simulink model "parent_model_v2"  (R2020b)
settings: Solver=VariableStepAuto  StartTime=0.0  StopTime=10.0  RelTol=1e-3
libraries: sdl_lib x14, nesl_utility x12, autolibmappedmotor x4, autolibdatasheetbattery x1, autolibshared x1
settings Model: Creator=True  LastModifiedBy=True

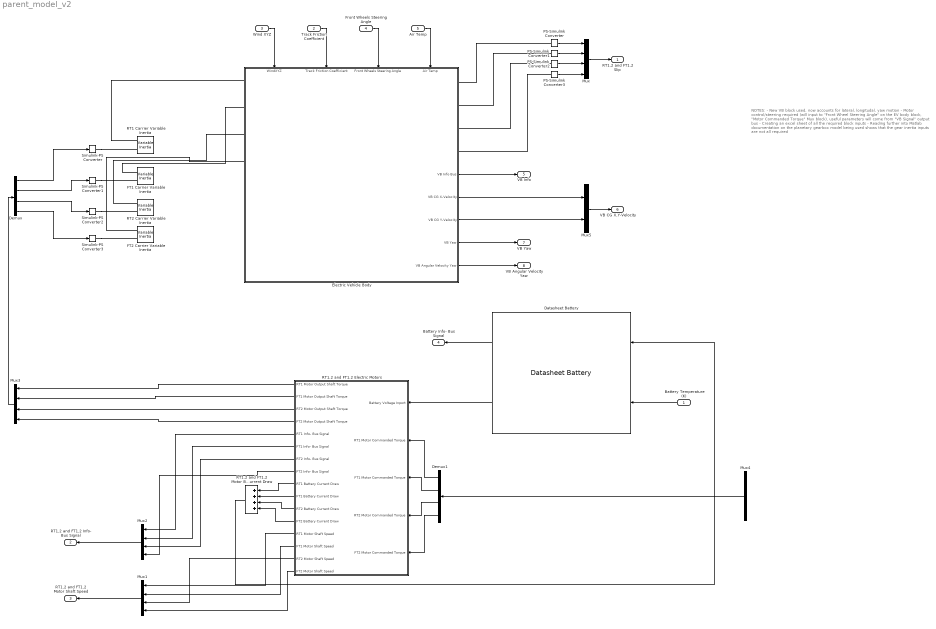
== system parent_model_v2 ==
  note: NOTES:
      | - New VB block used, now accounts for lateral, longitudal, yaw motion
      |
      | - Motor control/steering required (will input to "Front Wheel Steering Angle" on the EV body block, "Motor Commanded Torque" Mux block), useful parameters will come from "VB Signal" output bus
      |
      | - Creating an excel sheet of all the required block inputs
      |
      | - Reading further into Matlab documentation on the planetary gearbox model being used shows that the gear inertia inputs are not all required
  Battery Temperature (K) : Inport
  Track Friction Coefficient : Inport  Port=2
  Wind XYZ : Inport  Port=3
  Front Wheels Steering Angle : Inport  Port=4
  Air Temp : Inport  Port=5
  Datasheet Battery : autolibdatasheetbattery/Datasheet Battery  CapacityCtrl=Parameter  OutputVlt=Unfiltered  BattChargeMax=100  Em=[2.8 3.228 3.284 3.361 3.408 3.427 3.472 3.477 3.493 3.504 3.516 3.528 3.537 3.545 3.555 3.561 3.566 3.576 3.587 3.589 3.594 3.6 3.608 3.61 3.616 3.619 3.626 3.632 3.637 3.64 3.645 3.646 3.652 3.655 3.658 3.661 3.664 3.668 3.673 3.678 3.68 3.681 3.686 3.692 3.699 3.702 3.705 3.71 3.717 3.723 3.728 3.733 3.735 3.742 3.749 3.755 3.761 3.768 3.773 3.78 3.791 3.798 3.798 3.814 3.818 3.825 3.841 3.846 3.855 3.863 3.877 3.885 3.894 3.907 3.919 3.926 3.935 3.944 3.954 3.964 3.974 3.988 3.998 4.014 4.029 4.034 4.047 4.065 4.074 4.086 4.097 4.131 4.126 4.138 4.15 4.18 4.174 4.187 4.207 4.231 4.221]  CapLUTBp=[0 0.01 0.02 0.03 0.04 0.05 0.06 0.07 0.08 0.09 0.1 0.11 0.12 0.13 0.14 0.15 0.16 0.17 0.18 0.19 0.2 0.21 0.22 0.23 0.24 0.25 0.26 0.27 0.28 0.29 0.3 0.31 0.32 0.33 0.34 0.35 0.36 0.37 0.38 0.39 0.4 0.41 0.42 0.43 0.44 0.45 0.46 0.47 0.48 0.49 0.5 0.51 0.52 0.53 0.54 0.55 0.56 0.57 0.58 0.59 0.6 0.61 0.62 0.63 0.64 0.65 0.66 0.67 0.68 0.69 0.7 0.71 0.72 0.73 0.74 0.75 0.76 0.77 0.78 0.79 0.8 0.81 0.82 0.83 0.84 0.85 0.86 0.87 0.88 0.89 0.9 0.91 0.92 0.93 0.94 0.95 0.96 0.97 0.98 0.99 1]  RInt=[0.008846 0.009319 0.009027 0.00847 0.01032 0.01314;0.006389 0.006554 0.005553 0.005525 0.006043 0.007805;0.004364 0.004101 0.00406 0.003452 0.003846 0.004517;0.002031 0.002563 0.002532 0.00246 0.002716 0.003047;0.001443 0.001825 0.001795 0.001778 0.001924 0.002234;0.0005603 0.0007192 0.0006887 0.0007557 0.0007355 0.001014;0.001028 0.001338 0.001 0.001536 0.001546 0.002789]  BattTempBp=[243.1 253.1 263.1 273.1 283.1 298.1 313.1]  CapSOCBp=[0 0.2 0.4 0.6 0.8 1]  Ns=1  Np=1  BattCapInit=100  Tc=1/1000  Vinit=4.221  RefBlkName='autolibdatasheetbattery/Datasheet Battery'
      settings: SourceProductBaseCode=PW
  Demux : Demux
  Demux1 : Demux
  Electric Vehicle Body : Subsystem
      settings: PortSchema="{\"entries\":[{\"content\":{\"sides\":[{\"content\":{\"connectorIds\":[\"LConn1\",\"LConn2\",\"LConn3\",\"LConn4\",\"LConn5\",\"LConn6\",\"LConn7\",\"LConn8\"]},\"type\":\"ConnectorPlacement.EquallySpacedRectSide\",\"uuid\":\"3589ffd8-3282-449f-9f73-db5573b89272\"},{\"content\":{\"connectorIds\":[\"RConn1\",\"RConn2\",\"RConn3\",\"RConn4\",\"Out1\",\"Out2\",\"Out3\",\"Out4\",\"Out5\"],\"side\":\"RIGHT\"},\"type\":\"ConnectorPlacement.EquallySpacedRectSide\",\"uuid\":\"4bc75fc4-5a6d-4cdc-a1d8-7589f1bfd0e3\"},{\"content\":{\"connectorIds\":[\"In1\",\"In2\",\"In3\",\"In4\"],\"side\":\"TOP\"},\"type\":\"ConnectorPlacement.EquallySpacedRectSide\",\"uuid\":\"5582f31c-489d-4354-9c03-0beb1d144974\"},{\"content\":{\"connectorIds\":[],\"side\":\"BOTTOM\"},\"type\":\"ConnectorPlacement.EquallySpacedRectSide\",\"uuid\":\"e952a40a-921b-4756-bc3d-1bba2f446a83\"},{\"content\":{\"connectorIds\":[],\"side\":\"HIDDEN\"},\"type\":\"ConnectorPlacement.EquallySpacedRectSide\",\"uuid\":\"95051cab-6025-4def-8e94-855365c64cfc\"}]},\"type\":\"ConnectorPlacement.EquallySpacedConnector\",\"uuid\":\"f0af1aeb-7bbe-491f-85c8-fb0f3026e409\"}],\"packageUris\":[\"http://schema.mathworks.com/mf0/Connector/R2020b\"],\"version\":\"1.0\"}"
  FT1 Carrier Variable Inertia : sdl_lib/Inertias & Loads/Variable Inertia  minimum_inertia=0.1 kg*m^2  L_specify=off  L_priority=High  L=0 m^2*kg/s  L_nominal_specify=off  L_nominal_unit=m^2*kg/s  L_nominal_value=1
      settings: SourceProductBaseCode=LD  InternalSimscapePortConfiguration="{\"Bottom\":[],\"Left\":[{\"id\":\"I\",\"label\":\"\",\"type\":\"input\"},{\"id\":\"A\",\"label\":\"\",\"type\":\"foundation.mechanical.rotational.rotational\"}],\"Right\":[],\"Top\":[]}"
  FT2 Carrier Variable Inertia : sdl_lib/Inertias & Loads/Variable Inertia  minimum_inertia=0.1 kg*m^2  L_specify=off  L_priority=High  L=0 m^2*kg/s  L_nominal_specify=off  L_nominal_unit=m^2*kg/s  L_nominal_value=1
      settings: SourceProductBaseCode=LD  InternalSimscapePortConfiguration="{\"Bottom\":[],\"Left\":[{\"id\":\"I\",\"label\":\"\",\"type\":\"input\"},{\"id\":\"A\",\"label\":\"\",\"type\":\"foundation.mechanical.rotational.rotational\"}],\"Right\":[],\"Top\":[]}"
  Mux{,1..4} (5 alike) : Mux
  Mux5 : Mux  Inputs=2
  PS-Simulink Converter{,1..3} (4 alike) : nesl_utility/PS-Simulink Converter  PhysicalDomain=network_engine_domain  SubClassName=ps_output  LeftPortType=input  RightPortType=output  PseudoPeriodic=off  Frequencies=[]  Unit=inherit  AffineConversion=off
  RT1 Carrier Variable Inertia : sdl_lib/Inertias & Loads/Variable Inertia  minimum_inertia=0.1 kg*m^2  L_specify=off  L_priority=High  L=0 m^2*kg/s  L_nominal_specify=off  L_nominal_unit=m^2*kg/s  L_nominal_value=1
      settings: SourceProductBaseCode=LD  InternalSimscapePortConfiguration="{\"Bottom\":[],\"Left\":[{\"id\":\"I\",\"label\":\"\",\"type\":\"input\"},{\"id\":\"A\",\"label\":\"\",\"type\":\"foundation.mechanical.rotational.rotational\"}],\"Right\":[],\"Top\":[]}"
  RT1,2 and FT1,2 Electric Motors : Subsystem
  RT1,2 and FT1,2 Motor Battery Current Draw : Sum  Inputs=++++
  RT2 Carrier Variable Inertia : sdl_lib/Inertias & Loads/Variable Inertia  minimum_inertia=0.1 kg*m^2  L_specify=off  L_priority=High  L=0 m^2*kg/s  L_nominal_specify=off  L_nominal_unit=m^2*kg/s  L_nominal_value=1
      settings: SourceProductBaseCode=LD  InternalSimscapePortConfiguration="{\"Bottom\":[],\"Left\":[{\"id\":\"I\",\"label\":\"\",\"type\":\"input\"},{\"id\":\"A\",\"label\":\"\",\"type\":\"foundation.mechanical.rotational.rotational\"}],\"Right\":[],\"Top\":[]}"
  Simulink-PS Converter{,1..3} (4 alike) : nesl_utility/Simulink-PS Converter  PhysicalDomain=network_engine_domain  SubClassName=ps_input  LeftPortType=input  RightPortType=output  PseudoPeriodic=off  Frequencies=[]  NoiseDistribution=none  NoiseParameters=[]  Unit=1  AffineConversion=off  FilteringAndDerivatives=provide  SimscapeFilterOrder=1  InputFilterTimeConstant=0.001  UdotUserProvided=0
  RT1,2 and FT1,2 Slip : Outport
  RT1,2 and FT1,2 Info- Bus Signal : Outport  Port=2
  RT1,2 and FT1,2 Motor Shaft Speed : Outport  Port=3
  Battery Info- Bus Signal : Outport  Port=4
  VB Info : Outport  Port=5
  VB CG X,Y-Velocity : Outport  Port=6
  VB Yaw : Outport  Port=7
  VB Angular Velocity Yaw : Outport  Port=8
  wires:
  Datasheet Battery/2 -> RT1,2 and FT1,2 Electric Motors/1(Battery Voltage Inport)
  RT1,2 and FT1,2 Electric Motors/9(RT1 Battery Current Draw) -> RT1,2 and FT1,2 Motor Battery Current Draw/1
  RT1,2 and FT1,2 Electric Motors/10(FT1 Battery Current Draw) -> RT1,2 and FT1,2 Motor Battery Current Draw/2
  RT1,2 and FT1,2 Electric Motors/11(RT2 Battery Current Draw) -> RT1,2 and FT1,2 Motor Battery Current Draw/3
  RT1,2 and FT1,2 Electric Motors/12(FT2 Battery Current Draw) -> RT1,2 and FT1,2 Motor Battery Current Draw/4
  RT1,2 and FT1,2 Motor Battery Current Draw/1 -> Datasheet Battery/1
  Battery Temperature (K)/1 -> Datasheet Battery/2
  PS-Simulink Converter/1 -> Mux/1
  PS-Simulink Converter1/1 -> Mux/2
  PS-Simulink Converter2/1 -> Mux/3
  PS-Simulink Converter3/1 -> Mux/4
  Mux/1 -> RT1,2 and FT1,2 Slip/1
  RT1,2 and FT1,2 Electric Motors/5(RT1 Info- Bus Signal) -> Mux2/1
  RT1,2 and FT1,2 Electric Motors/6(FT1 Info- Bus Signal) -> Mux2/2
  RT1,2 and FT1,2 Electric Motors/7(RT2 Info- Bus Signal) -> Mux2/3
  RT1,2 and FT1,2 Electric Motors/8(FT2 Info- Bus Signal) -> Mux2/4
  RT1,2 and FT1,2 Electric Motors/13(RT1 Motor Shaft Speed) -> Mux1/1
  RT1,2 and FT1,2 Electric Motors/14(FT1 Motor Shaft Speed) -> Mux1/2
  RT1,2 and FT1,2 Electric Motors/15(RT2 Motor Shaft Speed) -> Mux1/3
  RT1,2 and FT1,2 Electric Motors/16(FT2 Motor Shaft Speed) -> Mux1/4
  Mux2/1 -> RT1,2 and FT1,2 Info- Bus Signal/1
  Mux1/1 -> RT1,2 and FT1,2 Motor Shaft Speed/1
  Datasheet Battery/1 -> Battery Info- Bus Signal/1
  Demux/1 -> Simulink-PS Converter/1
  Demux/4 -> Simulink-PS Converter3/1
  Demux/3 -> Simulink-PS Converter2/1
  Demux/2 -> Simulink-PS Converter1/1
  RT1,2 and FT1,2 Electric Motors/1(RT1 Motor Output Shaft Torque) -> Mux3/1
  RT1,2 and FT1,2 Electric Motors/2(FT1 Motor Output Shaft Torque) -> Mux3/2
  RT1,2 and FT1,2 Electric Motors/3(RT2 Motor Output Shaft Torque) -> Mux3/3
  RT1,2 and FT1,2 Electric Motors/4(FT2 Motor Output Shaft Torque) -> Mux3/4
  Mux3/1 -> Demux/1
  Demux1/1 -> RT1,2 and FT1,2 Electric Motors/2(RT1 Motor Commanded Torque)
  Demux1/2 -> RT1,2 and FT1,2 Electric Motors/3("FT1 Motor Commanded Torque ")
  Demux1/3 -> RT1,2 and FT1,2 Electric Motors/4(RT2 Motor Commanded Torque)
  Demux1/4 -> RT1,2 and FT1,2 Electric Motors/5(FT2 Motor Commanded Torque)
  Mux4/1 -> Demux1/1
  Electric Vehicle Body/1(VB Info Bus) -> VB Info/1
  Electric Vehicle Body/2("VB CG X-Velocity ") -> Mux5/1
  Electric Vehicle Body/3(VB CG Y-Velocity) -> Mux5/2
  Mux5/1 -> VB CG X,Y-Velocity/1
  Electric Vehicle Body/4(VB Yaw) -> VB Yaw/1
  Electric Vehicle Body/5(VB Angular Velocity Yaw) -> VB Angular Velocity Yaw/1
  Track Friction Coefficient/1 -> Electric Vehicle Body/2(Track Friction Coefficient)
  Wind XYZ/1 -> Electric Vehicle Body/1(WindXYZ)
  Front Wheels Steering Angle/1 -> Electric Vehicle Body/3(Front Wheels Steering Angle)
  Air Temp/1 -> Electric Vehicle Body/4(Air Temp)
  connections:
  Simulink-PS Converter1/RConn1 -- FT1 Carrier Variable Inertia/LConn1
  Simulink-PS Converter2/RConn1 -- RT2 Carrier Variable Inertia/LConn1
  Simulink-PS Converter/RConn1 -- RT1 Carrier Variable Inertia/LConn1
  Simulink-PS Converter3/RConn1 -- FT2 Carrier Variable Inertia/LConn1
  PS-Simulink Converter/LConn1 -- Electric Vehicle Body/RConn1
  PS-Simulink Converter1/LConn1 -- Electric Vehicle Body/RConn2
  Electric Vehicle Body/LConn1 -- RT1 Carrier Variable Inertia/LConn2
  PS-Simulink Converter2/LConn1 -- Electric Vehicle Body/RConn3
  PS-Simulink Converter3/LConn1 -- Electric Vehicle Body/RConn4
  FT1 Carrier Variable Inertia/LConn2 -- Electric Vehicle Body/LConn2
  RT2 Carrier Variable Inertia/LConn2 -- Electric Vehicle Body/LConn3
  FT2 Carrier Variable Inertia/LConn2 -- Electric Vehicle Body/LConn4

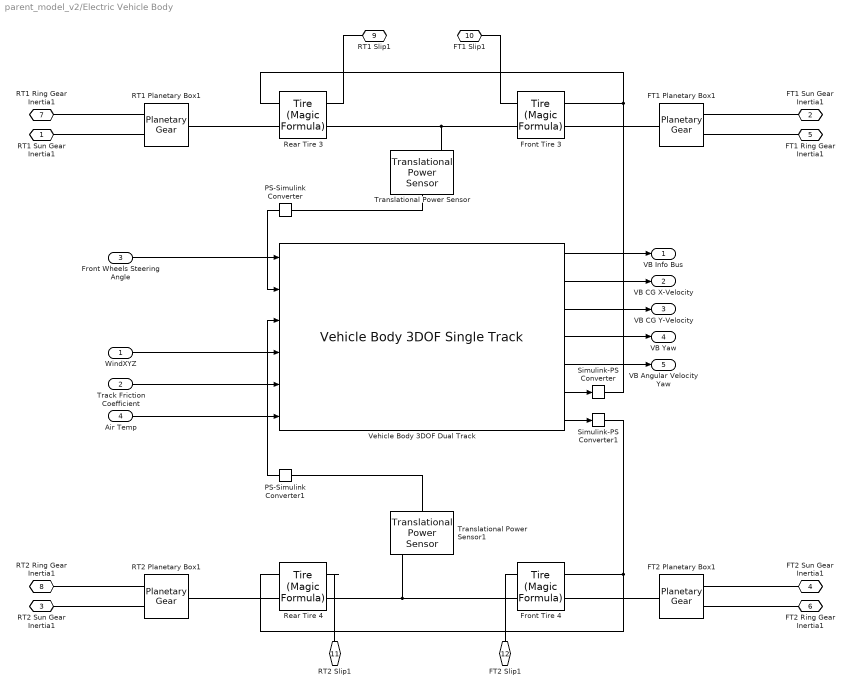
== system parent_model_v2/Electric Vehicle Body ==
  WindXYZ : Inport
  Track Friction Coefficient : Inport  Port=2
  Front Wheels Steering Angle : Inport  Port=3
  Air Temp : Inport  Port=4
  FT1 Planetary Box1 : sdl_lib/Gears/Planetary Gear  rs_ratio=2  friction_model=sdl.enum.gear_friction.none  mu_visc=[0, 0] N*m/(rad/s)  efficiency=[.96, .98]  temperature_TLU=[280, 300, 320] K  efficiency_sp_TLU=[.95, .9, .85]  efficiency_rp_TLU=[.95, .9, .85]  pwr_thr=[.001, .001] W  thermal_mass=50 J/K  T_init=300 K  model_inertia=simscape.enum.onoff.off  planet_inertia=0.001 kg*m^2
      settings: SourceProductBaseCode=LD
  FT2 Planetary Box1 : sdl_lib/Gears/Planetary Gear  rs_ratio=2  friction_model=sdl.enum.gear_friction.none  mu_visc=[0, 0] N*m/(rad/s)  efficiency=[.96, .98]  temperature_TLU=[280, 300, 320] K  efficiency_sp_TLU=[.95, .9, .85]  efficiency_rp_TLU=[.95, .9, .85]  pwr_thr=[.001, .001] W  thermal_mass=50 J/K  T_init=300 K  model_inertia=simscape.enum.onoff.off  planet_inertia=0.001 kg*m^2
      settings: SourceProductBaseCode=LD
  Front Tire 3 : sdl_lib/Tires & Vehicles/Tire (Magic Formula)  parameterization=sdl.enum.magic_tire_model.peak  F_z1=3000 N  F_x1=3500 N  kappa1=10  B_m=10  C_m=1.9  D_m=1  E_m=0.97  fz0=4000 N  p_Cx=1.685  p_Dx=[1.21, -.037]  p_Ex=[.344, .095, -.02, 0]  p_Kx=[21.51, -.163, .245]  p_Hx=[-.002, .002]  p_Vx=[0, 0]  v_tr_thr=0.1 m/s  r_e=0.3 m  model_compliance=0  stiffness=1e6 N/m  damping=1000 N/(m/s)  model_inertia=0  inertia=1 kg*m^2  initial_velocity=0 rad/s  model_resistance=0  resistance_model=1  coeff=0.015  p_tire=250e3 Pa  alpha=-0.003  beta=0.97  coeff_a=84e-4  coeff_b=6.2e-4 s/m  coeff_c=1.6e-4 s^2/m^2  v_thr=0.001 m/s
  Front Tire 4 : sdl_lib/Tires & Vehicles/Tire (Magic Formula)  parameterization=sdl.enum.magic_tire_model.peak  F_z1=3000 N  F_x1=3500 N  kappa1=10  B_m=10  C_m=1.9  D_m=1  E_m=0.97  fz0=4000 N  p_Cx=1.685  p_Dx=[1.21, -.037]  p_Ex=[.344, .095, -.02, 0]  p_Kx=[21.51, -.163, .245]  p_Hx=[-.002, .002]  p_Vx=[0, 0]  v_tr_thr=0.1 m/s  r_e=0.3 m  model_compliance=0  stiffness=1e6 N/m  damping=1000 N/(m/s)  model_inertia=0  inertia=1 kg*m^2  initial_velocity=0 rad/s  model_resistance=0  resistance_model=1  coeff=0.015  p_tire=250e3 Pa  alpha=-0.003  beta=0.97  coeff_a=84e-4  coeff_b=6.2e-4 s/m  coeff_c=1.6e-4 s^2/m^2  v_thr=0.001 m/s
  PS-Simulink Converter : nesl_utility/PS-Simulink Converter  PhysicalDomain=network_engine_domain  SubClassName=ps_output  LeftPortType=input  RightPortType=output  PseudoPeriodic=off  Frequencies=[]  Unit=inherit  AffineConversion=off
  PS-Simulink Converter1 : nesl_utility/PS-Simulink Converter  PhysicalDomain=network_engine_domain  SubClassName=ps_output  LeftPortType=input  RightPortType=output  PseudoPeriodic=off  Frequencies=[]  Unit=inherit  AffineConversion=off
  RT1 Planetary Box1 : sdl_lib/Gears/Planetary Gear  rs_ratio=2  friction_model=sdl.enum.gear_friction.none  mu_visc=[0, 0] N*m/(rad/s)  efficiency=[.96, .98]  temperature_TLU=[280, 300, 320] K  efficiency_sp_TLU=[.95, .9, .85]  efficiency_rp_TLU=[.95, .9, .85]  pwr_thr=[.001, .001] W  thermal_mass=50 J/K  T_init=300 K  model_inertia=simscape.enum.onoff.off  planet_inertia=0.001 kg*m^2
      settings: SourceProductBaseCode=LD
  RT2 Planetary Box1 : sdl_lib/Gears/Planetary Gear  rs_ratio=2  friction_model=sdl.enum.gear_friction.none  mu_visc=[0, 0] N*m/(rad/s)  efficiency=[.96, .98]  temperature_TLU=[280, 300, 320] K  efficiency_sp_TLU=[.95, .9, .85]  efficiency_rp_TLU=[.95, .9, .85]  pwr_thr=[.001, .001] W  thermal_mass=50 J/K  T_init=300 K  model_inertia=simscape.enum.onoff.off  planet_inertia=0.001 kg*m^2
      settings: SourceProductBaseCode=LD
  Rear Tire 3 : sdl_lib/Tires & Vehicles/Tire (Magic Formula)  parameterization=sdl.enum.magic_tire_model.peak  F_z1=3000 N  F_x1=3500 N  kappa1=10  B_m=10  C_m=1.9  D_m=1  E_m=0.97  fz0=4000 N  p_Cx=1.685  p_Dx=[1.21, -.037]  p_Ex=[.344, .095, -.02, 0]  p_Kx=[21.51, -.163, .245]  p_Hx=[-.002, .002]  p_Vx=[0, 0]  v_tr_thr=0.1 m/s  r_e=0.3 m  model_compliance=0  stiffness=1e6 N/m  damping=1000 N/(m/s)  model_inertia=0  inertia=1 kg*m^2  initial_velocity=0 rad/s  model_resistance=0  resistance_model=1  coeff=0.015  p_tire=250e3 Pa  alpha=-0.003  beta=0.97  coeff_a=84e-4  coeff_b=6.2e-4 s/m  coeff_c=1.6e-4 s^2/m^2  v_thr=0.001 m/s
  Rear Tire 4 : sdl_lib/Tires & Vehicles/Tire (Magic Formula)  parameterization=sdl.enum.magic_tire_model.peak  F_z1=3000 N  F_x1=3500 N  kappa1=10  B_m=10  C_m=1.9  D_m=1  E_m=0.97  fz0=4000 N  p_Cx=1.685  p_Dx=[1.21, -.037]  p_Ex=[.344, .095, -.02, 0]  p_Kx=[21.51, -.163, .245]  p_Hx=[-.002, .002]  p_Vx=[0, 0]  v_tr_thr=0.1 m/s  r_e=0.3 m  model_compliance=0  stiffness=1e6 N/m  damping=1000 N/(m/s)  model_inertia=0  inertia=1 kg*m^2  initial_velocity=0 rad/s  model_resistance=0  resistance_model=1  coeff=0.015  p_tire=250e3 Pa  alpha=-0.003  beta=0.97  coeff_a=84e-4  coeff_b=6.2e-4 s/m  coeff_c=1.6e-4 s^2/m^2  v_thr=0.001 m/s
  Simulink-PS Converter : nesl_utility/Simulink-PS Converter  PhysicalDomain=network_engine_domain  SubClassName=ps_input  LeftPortType=input  RightPortType=output  PseudoPeriodic=off  Frequencies=[]  NoiseDistribution=none  NoiseParameters=[]  Unit=1  AffineConversion=off  FilteringAndDerivatives=provide  SimscapeFilterOrder=1  InputFilterTimeConstant=0.001  UdotUserProvided=0
  Simulink-PS Converter1 : nesl_utility/Simulink-PS Converter  PhysicalDomain=network_engine_domain  SubClassName=ps_input  LeftPortType=input  RightPortType=output  PseudoPeriodic=off  Frequencies=[]  NoiseDistribution=none  NoiseParameters=[]  Unit=1  AffineConversion=off  FilteringAndDerivatives=provide  SimscapeFilterOrder=1  InputFilterTimeConstant=0.001  UdotUserProvided=0
  Translational Power Sensor : sdl_lib/Sensors/Translational Power Sensor  measurement_type=1  averaging_period=1 s  max_frequency=1000 Hz
      settings: SourceProductBaseCode=LD  InternalSimscapePortConfiguration="{\"Bottom\":[],\"Left\":[{\"id\":\"S\",\"label\":\"S\",\"type\":\"foundation.mechanical.translational.translational\"},{\"id\":\"R\",\"label\":\"R\",\"type\":\"foundation.mechanical.translational.translational\"},{\"id\":\"C\",\"label\":\"C\",\"type\":\"foundation.mechanical.translational.translational\"}],\"Right\":[{\"id\":\"P\",\"label\":\"P\",\"type\":\"output\"}],\"Top\":[]}"
  Translational Power Sensor1 : sdl_lib/Sensors/Translational Power Sensor  measurement_type=1  averaging_period=1 s  max_frequency=1000 Hz
      settings: SourceProductBaseCode=LD  InternalSimscapePortConfiguration="{\"Bottom\":[],\"Left\":[{\"id\":\"S\",\"label\":\"S\",\"type\":\"foundation.mechanical.translational.translational\"},{\"id\":\"R\",\"label\":\"R\",\"type\":\"foundation.mechanical.translational.translational\"},{\"id\":\"C\",\"label\":\"C\",\"type\":\"foundation.mechanical.translational.translational\"}],\"Right\":[{\"id\":\"P\",\"label\":\"P\",\"type\":\"output\"}],\"Top\":[]}"
  Vehicle Body 3DOF Dual Track : autolibshared/Vehicle Body 3DOF Single Track  trackMode=Dual  inputMode=External longitudinal forces  frontSteerMode=on  rearSteerMode=off  windMode=on  muMode=on  extFMode=off  extMMode=off  htchFMode=off  htchMMode=off  extXo=off  extpsio=off  extxdoto=off  extro=off  extYo=off  extTamb=on  extydoto=off  aMode=2  NF=2  NR=2  m=2000  a=1.4  b=1.6  h=0.35  dh=1  hh=0.2  X_o=0  xdot_o=0  CalphaMode=off  sigmaMode=on  d=0  hl=0  w=[1.4,1.4]  Cy_f=12e3  Cy_r=11e3  sigma_f=.1  sigma_r=.1  alpha_f_brk=[-.1 .1]  Cy_f_data=[-9e3 9e3]  alpha_r_brk=[-.1 .1]  Cy_r_data=[-9e3 9e3]  Y_o=0  ydot_o=0  Izz=4000  psi_o=0  r_o=0  Af=2  Cd=.3  Cl=.1  Cpm=.1  beta_w=[0:0.01:0.3]  Cs=[0:0.03:0.9]  Cym=[0:0.01:0.3]  Pabs=101325  Tair=273  g=9.81  mu=1  xdot_tol=.01  Fznom=5000  Fxtire_sat=7e4  Fytire_sat=7e4  longOff=0  latOff=0  vertOff=0  wrapAng=off
      settings: SourceProductBaseCode=PW,MT,UV,VE,VP
  RT1 Sun Gear Inertia1 : PMIOPort  Side=Left
  FT1 Sun Gear Inertia1 : PMIOPort  Port=2  Side=Left
  RT2 Sun Gear Inertia1 : PMIOPort  Port=3  Side=Left
  FT2 Sun Gear Inertia1 : PMIOPort  Port=4  Side=Left
  FT1 Ring Gear Inertia1 : PMIOPort  Port=5  Side=Left
  FT2 Ring Gear Inertia1 : PMIOPort  Port=6  Side=Left
  RT1 Ring Gear Inertia1 : PMIOPort  Port=7  Side=Left
  RT2 Ring Gear Inertia1 : PMIOPort  Port=8  Side=Left
  RT1 Slip1 : PMIOPort  Port=9  Side=Right
  FT1 Slip1 : PMIOPort  Port=10  Side=Right
  RT2 Slip1 : PMIOPort  Port=11  Side=Right
  FT2 Slip1 : PMIOPort  Port=12  Side=Right
  VB Info Bus : Outport
  "VB CG X-Velocity " : Outport  Port=2
  VB CG Y-Velocity : Outport  Port=3
  VB Yaw : Outport  Port=4
  VB Angular Velocity Yaw : Outport  Port=5
  wires:
  PS-Simulink Converter/1 -> Vehicle Body 3DOF Dual Track/2
  PS-Simulink Converter1/1 -> Vehicle Body 3DOF Dual Track/3
  Vehicle Body 3DOF Dual Track/6 -> Simulink-PS Converter/1
  Vehicle Body 3DOF Dual Track/7 -> Simulink-PS Converter1/1
  Air Temp/1 -> Vehicle Body 3DOF Dual Track/6
  Front Wheels Steering Angle/1 -> Vehicle Body 3DOF Dual Track/1
  Track Friction Coefficient/1 -> Vehicle Body 3DOF Dual Track/5
  WindXYZ/1 -> Vehicle Body 3DOF Dual Track/4
  Vehicle Body 3DOF Dual Track/1 -> VB Info Bus/1
  Vehicle Body 3DOF Dual Track/2 -> "VB CG X-Velocity "/1
  Vehicle Body 3DOF Dual Track/3 -> VB CG Y-Velocity/1
  Vehicle Body 3DOF Dual Track/4 -> VB Yaw/1
  Vehicle Body 3DOF Dual Track/5 -> VB Angular Velocity Yaw/1
  connections:
  Rear Tire 4/RConn2 -- Translational Power Sensor1/LConn1 -- Front Tire 4/RConn2
  RT1 Ring Gear Inertia1/RConn1 -- RT1 Planetary Box1/RConn1
  FT2 Ring Gear Inertia1/RConn1 -- FT2 Planetary Box1/RConn1
  RT2 Ring Gear Inertia1/RConn1 -- RT2 Planetary Box1/RConn1
  Rear Tire 4/LConn2 -- RT2 Planetary Box1/LConn1
  FT2 Sun Gear Inertia1/RConn1 -- FT2 Planetary Box1/RConn2
  Rear Tire 4/RConn1 -- RT2 Slip1/RConn1
  Front Tire 3/RConn1 -- FT1 Slip1/RConn1
  RT2 Sun Gear Inertia1/RConn1 -- RT2 Planetary Box1/RConn2
  Rear Tire 3/RConn1 -- RT1 Slip1/RConn1
  FT1 Ring Gear Inertia1/RConn1 -- FT1 Planetary Box1/RConn1
  Front Tire 4/RConn1 -- FT2 Slip1/RConn1
  FT1 Planetary Box1/LConn1 -- Front Tire 3/LConn2
  Front Tire 4/LConn2 -- FT2 Planetary Box1/LConn1
  RT1 Sun Gear Inertia1/RConn1 -- RT1 Planetary Box1/RConn2
  RT1 Planetary Box1/LConn1 -- Rear Tire 3/LConn2
  FT1 Sun Gear Inertia1/RConn1 -- FT1 Planetary Box1/RConn2
  PS-Simulink Converter/LConn1 -- Translational Power Sensor/RConn1
  Rear Tire 3/RConn2 -- Front Tire 3/RConn2 -- Translational Power Sensor/LConn1
  PS-Simulink Converter1/LConn1 -- Translational Power Sensor1/RConn1
  Simulink-PS Converter/RConn1 -- Rear Tire 3/LConn1 -- Front Tire 3/LConn1
  Simulink-PS Converter1/RConn1 -- Rear Tire 4/LConn1 -- Front Tire 4/LConn1

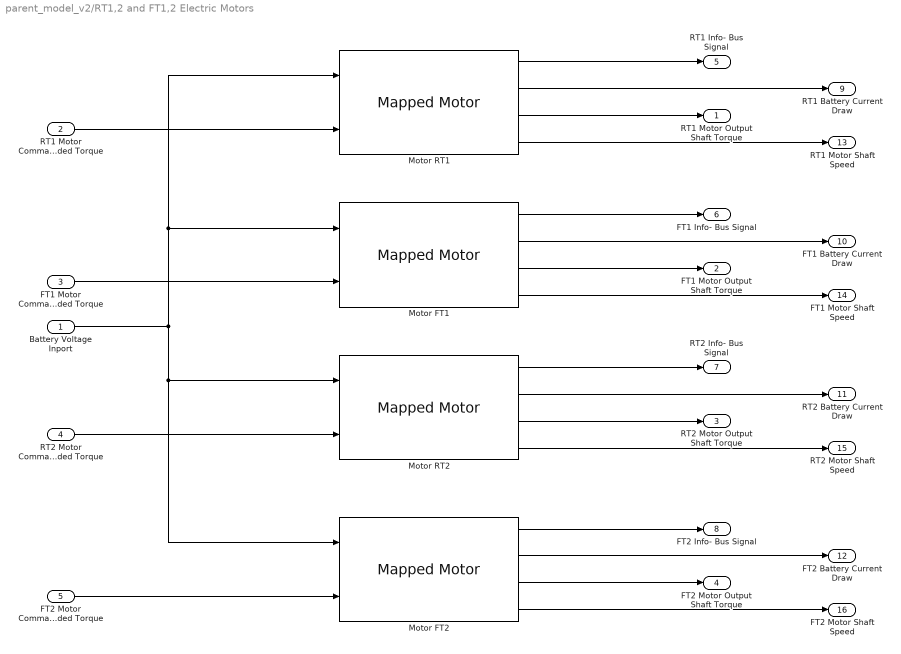
== system parent_model_v2/RT1,2 and FT1,2 Electric Motors ==
  Battery Voltage Inport : Inport
  RT1 Motor Commanded Torque : Inport  Port=2
  "FT1 Motor Commanded Torque " : Inport  Port=3
  RT2 Motor Commanded Torque : Inport  Port=4
  FT2 Motor Commanded Torque : Inport  Port=5
  Motor FT1 : autolibmappedmotor/Mapped Motor  port_config=Torque  param_by=Tabulated torque-speed envelope  w_t=[ 0 375 750 800 ]  T_t=[0.09 0.08 0.07 0]  torque_max=.1  power_max=30  Tc=0.02  param_loss=Single efficiency measurement  eff=100  w_eff=375  T_eff=0.08  Piron=0  Pbase=0  w_eff_bp=[-8000 -4000 0 4000 8000]  T_eff_bp=[0 0.03 0.06 0.09]  Temp_eff_bp=[233.15 293.15 373.15]  losses_table=[1.49 1.67 2.21 3.10; 0.42 0.69 1.14 2.03; 0.06 0.24 0.78 1.68; 0.42 0.69 1.14 2.03; 1.49 1.67 2.21 3.10]  losses_table_3d=cat(3,[1.49 1.67 2.21 3.10; 0.42 0.69 1.14 2.03; 0.06 0.24 0.78 1.68; 0.42 0.69 1.14 2.03; 1.49 1.67 2.21 3.10],[1.49 1.67 2.21 3.10; 0.42 0.69 1.14 2.03; 0.06 0.24 0.78 1.68; 0.42 0.69 1.14 2.03; 1.49 1.67 2.21 3.10],[1.49 1.67 2.21 3.10; 0.42 0.69 1.14 2.03; 0.06 0.24 0.78 1.68; 0.42 0.69 1.14 2.03; 1.49 1.67 2.21 3.10])  efficiency_table=[95 95 95 95; 95 95 95 95; 95 95 95 95; 95 95 95 95; 95 95 95 95]  efficiency_table_3d=cat(3,[95 95 95 95; 95 95 95 95; 95 95 95 95; 95 95 95 95; 95 95 95 95],[95 95 95 95; 95 95 95 95; 95 95 95 95; 95 95 95 95; 95 95 95 95],[95 95 95 95; 95 95 95 95; 95 95 95 95; 95 95 95 95; 95 95 95 95])  J=5e-6  b=1e-5  omega_o=0  T_t_extended=[0 0.07 0.08 0.09 0.08 0.07 0]  w_t_extended=[-800 -750 -375 0 375 750 800]  KLossIron=0  KLossCopper=0  x_w_eff_vec=[-8000 -4000 0 4000 8000]  x_T_eff_vec=[-0.09 -0.06 -0.03 0 0.03 0.06 0.09]  x_tmp_eff_vec=[-0.09 -0.06 -0.03 0 0.03 0.06 0.09]  x_losses_mat=[3.1 2.21 1.67 1.49 1.67 2.21 3.1;2.03 1.14 0.69 0.42 0.69 1.14 2.03;1.68 0.78 0.24 0.06 0.24 0.78 1.68;2.03 1.14 0.69 0.42 0.69 1.14 2.03;3.1 2.21 1.67 1.49 1.67 2.21 3.1]  x_losses_mat_3d=[37.8947368421052 25.2631578947368 12.6315789473684 0 12 24 36;18.9473684210526 12.6315789473684 6.3157894736842 0 5.99999999999999 12 18;0 0 0 0 0 0 0;18 12 5.99999999999999 0 6.3157894736842 12.6315789473684 18.9473684210526;36 24 12 0 12.6315789473684 25.2631578947368 37.8947368421052]  CalLossMapData={}  CalLossWithTempMapData={}  aMode=1  RefBlkName='autolibmappedmotor/Mapped Motor'
      settings: SourceProductBaseCode=PW,MT,UV,VE,VP
  Motor FT2 : autolibmappedmotor/Mapped Motor  port_config=Torque  param_by=Tabulated torque-speed envelope  w_t=[ 0 375 750 800 ]  T_t=[0.09 0.08 0.07 0]  torque_max=.1  power_max=30  Tc=0.02  param_loss=Single efficiency measurement  eff=100  w_eff=375  T_eff=0.08  Piron=0  Pbase=0  w_eff_bp=[-8000 -4000 0 4000 8000]  T_eff_bp=[0 0.03 0.06 0.09]  Temp_eff_bp=[233.15 293.15 373.15]  losses_table=[1.49 1.67 2.21 3.10; 0.42 0.69 1.14 2.03; 0.06 0.24 0.78 1.68; 0.42 0.69 1.14 2.03; 1.49 1.67 2.21 3.10]  losses_table_3d=cat(3,[1.49 1.67 2.21 3.10; 0.42 0.69 1.14 2.03; 0.06 0.24 0.78 1.68; 0.42 0.69 1.14 2.03; 1.49 1.67 2.21 3.10],[1.49 1.67 2.21 3.10; 0.42 0.69 1.14 2.03; 0.06 0.24 0.78 1.68; 0.42 0.69 1.14 2.03; 1.49 1.67 2.21 3.10],[1.49 1.67 2.21 3.10; 0.42 0.69 1.14 2.03; 0.06 0.24 0.78 1.68; 0.42 0.69 1.14 2.03; 1.49 1.67 2.21 3.10])  efficiency_table=[95 95 95 95; 95 95 95 95; 95 95 95 95; 95 95 95 95; 95 95 95 95]  efficiency_table_3d=cat(3,[95 95 95 95; 95 95 95 95; 95 95 95 95; 95 95 95 95; 95 95 95 95],[95 95 95 95; 95 95 95 95; 95 95 95 95; 95 95 95 95; 95 95 95 95],[95 95 95 95; 95 95 95 95; 95 95 95 95; 95 95 95 95; 95 95 95 95])  J=5e-6  b=1e-5  omega_o=0  T_t_extended=[0 0.07 0.08 0.09 0.08 0.07 0]  w_t_extended=[-800 -750 -375 0 375 750 800]  KLossIron=0  KLossCopper=0  x_w_eff_vec=[-8000 -4000 0 4000 8000]  x_T_eff_vec=[-0.09 -0.06 -0.03 0 0.03 0.06 0.09]  x_tmp_eff_vec=[-0.09 -0.06 -0.03 0 0.03 0.06 0.09]  x_losses_mat=[3.1 2.21 1.67 1.49 1.67 2.21 3.1;2.03 1.14 0.69 0.42 0.69 1.14 2.03;1.68 0.78 0.24 0.06 0.24 0.78 1.68;2.03 1.14 0.69 0.42 0.69 1.14 2.03;3.1 2.21 1.67 1.49 1.67 2.21 3.1]  x_losses_mat_3d=[37.8947368421052 25.2631578947368 12.6315789473684 0 12 24 36;18.9473684210526 12.6315789473684 6.3157894736842 0 5.99999999999999 12 18;0 0 0 0 0 0 0;18 12 5.99999999999999 0 6.3157894736842 12.6315789473684 18.9473684210526;36 24 12 0 12.6315789473684 25.2631578947368 37.8947368421052]  CalLossMapData={}  CalLossWithTempMapData={}  aMode=1  RefBlkName='autolibmappedmotor/Mapped Motor'
      settings: SourceProductBaseCode=PW,MT,UV,VE,VP
  Motor RT1 : autolibmappedmotor/Mapped Motor  port_config=Torque  param_by=Tabulated torque-speed envelope  w_t=[ 0 375 750 800 ]  T_t=[0.09 0.08 0.07 0]  torque_max=.1  power_max=30  Tc=0.02  param_loss=Single efficiency measurement  eff=100  w_eff=375  T_eff=0.08  Piron=0  Pbase=0  w_eff_bp=[-8000 -4000 0 4000 8000]  T_eff_bp=[0 0.03 0.06 0.09]  Temp_eff_bp=[233.15 293.15 373.15]  losses_table=[1.49 1.67 2.21 3.10; 0.42 0.69 1.14 2.03; 0.06 0.24 0.78 1.68; 0.42 0.69 1.14 2.03; 1.49 1.67 2.21 3.10]  losses_table_3d=cat(3,[1.49 1.67 2.21 3.10; 0.42 0.69 1.14 2.03; 0.06 0.24 0.78 1.68; 0.42 0.69 1.14 2.03; 1.49 1.67 2.21 3.10],[1.49 1.67 2.21 3.10; 0.42 0.69 1.14 2.03; 0.06 0.24 0.78 1.68; 0.42 0.69 1.14 2.03; 1.49 1.67 2.21 3.10],[1.49 1.67 2.21 3.10; 0.42 0.69 1.14 2.03; 0.06 0.24 0.78 1.68; 0.42 0.69 1.14 2.03; 1.49 1.67 2.21 3.10])  efficiency_table=[95 95 95 95; 95 95 95 95; 95 95 95 95; 95 95 95 95; 95 95 95 95]  efficiency_table_3d=cat(3,[95 95 95 95; 95 95 95 95; 95 95 95 95; 95 95 95 95; 95 95 95 95],[95 95 95 95; 95 95 95 95; 95 95 95 95; 95 95 95 95; 95 95 95 95],[95 95 95 95; 95 95 95 95; 95 95 95 95; 95 95 95 95; 95 95 95 95])  J=5e-6  b=1e-5  omega_o=0  T_t_extended=[0 0.07 0.08 0.09 0.08 0.07 0]  w_t_extended=[-800 -750 -375 0 375 750 800]  KLossIron=0  KLossCopper=0  x_w_eff_vec=[-8000 -4000 0 4000 8000]  x_T_eff_vec=[-0.09 -0.06 -0.03 0 0.03 0.06 0.09]  x_tmp_eff_vec=[-0.09 -0.06 -0.03 0 0.03 0.06 0.09]  x_losses_mat=[3.1 2.21 1.67 1.49 1.67 2.21 3.1;2.03 1.14 0.69 0.42 0.69 1.14 2.03;1.68 0.78 0.24 0.06 0.24 0.78 1.68;2.03 1.14 0.69 0.42 0.69 1.14 2.03;3.1 2.21 1.67 1.49 1.67 2.21 3.1]  x_losses_mat_3d=[37.8947368421052 25.2631578947368 12.6315789473684 0 12 24 36;18.9473684210526 12.6315789473684 6.3157894736842 0 5.99999999999999 12 18;0 0 0 0 0 0 0;18 12 5.99999999999999 0 6.3157894736842 12.6315789473684 18.9473684210526;36 24 12 0 12.6315789473684 25.2631578947368 37.8947368421052]  CalLossMapData={}  CalLossWithTempMapData={}  aMode=1  RefBlkName='autolibmappedmotor/Mapped Motor'
      settings: SourceProductBaseCode=PW,MT,UV,VE,VP
  Motor RT2 : autolibmappedmotor/Mapped Motor  port_config=Torque  param_by=Tabulated torque-speed envelope  w_t=[ 0 375 750 800 ]  T_t=[0.09 0.08 0.07 0]  torque_max=.1  power_max=30  Tc=0.02  param_loss=Single efficiency measurement  eff=100  w_eff=375  T_eff=0.08  Piron=0  Pbase=0  w_eff_bp=[-8000 -4000 0 4000 8000]  T_eff_bp=[0 0.03 0.06 0.09]  Temp_eff_bp=[233.15 293.15 373.15]  losses_table=[1.49 1.67 2.21 3.10; 0.42 0.69 1.14 2.03; 0.06 0.24 0.78 1.68; 0.42 0.69 1.14 2.03; 1.49 1.67 2.21 3.10]  losses_table_3d=cat(3,[1.49 1.67 2.21 3.10; 0.42 0.69 1.14 2.03; 0.06 0.24 0.78 1.68; 0.42 0.69 1.14 2.03; 1.49 1.67 2.21 3.10],[1.49 1.67 2.21 3.10; 0.42 0.69 1.14 2.03; 0.06 0.24 0.78 1.68; 0.42 0.69 1.14 2.03; 1.49 1.67 2.21 3.10],[1.49 1.67 2.21 3.10; 0.42 0.69 1.14 2.03; 0.06 0.24 0.78 1.68; 0.42 0.69 1.14 2.03; 1.49 1.67 2.21 3.10])  efficiency_table=[95 95 95 95; 95 95 95 95; 95 95 95 95; 95 95 95 95; 95 95 95 95]  efficiency_table_3d=cat(3,[95 95 95 95; 95 95 95 95; 95 95 95 95; 95 95 95 95; 95 95 95 95],[95 95 95 95; 95 95 95 95; 95 95 95 95; 95 95 95 95; 95 95 95 95],[95 95 95 95; 95 95 95 95; 95 95 95 95; 95 95 95 95; 95 95 95 95])  J=5e-6  b=1e-5  omega_o=0  T_t_extended=[0 0.07 0.08 0.09 0.08 0.07 0]  w_t_extended=[-800 -750 -375 0 375 750 800]  KLossIron=0  KLossCopper=0  x_w_eff_vec=[-8000 -4000 0 4000 8000]  x_T_eff_vec=[-0.09 -0.06 -0.03 0 0.03 0.06 0.09]  x_tmp_eff_vec=[-0.09 -0.06 -0.03 0 0.03 0.06 0.09]  x_losses_mat=[3.1 2.21 1.67 1.49 1.67 2.21 3.1;2.03 1.14 0.69 0.42 0.69 1.14 2.03;1.68 0.78 0.24 0.06 0.24 0.78 1.68;2.03 1.14 0.69 0.42 0.69 1.14 2.03;3.1 2.21 1.67 1.49 1.67 2.21 3.1]  x_losses_mat_3d=[37.8947368421052 25.2631578947368 12.6315789473684 0 12 24 36;18.9473684210526 12.6315789473684 6.3157894736842 0 5.99999999999999 12 18;0 0 0 0 0 0 0;18 12 5.99999999999999 0 6.3157894736842 12.6315789473684 18.9473684210526;36 24 12 0 12.6315789473684 25.2631578947368 37.8947368421052]  CalLossMapData={}  CalLossWithTempMapData={}  aMode=1  RefBlkName='autolibmappedmotor/Mapped Motor'
      settings: SourceProductBaseCode=PW,MT,UV,VE,VP
  RT1 Motor Output Shaft Torque : Outport
  FT1 Motor Output Shaft Torque : Outport  Port=2
  RT2 Motor Output Shaft Torque : Outport  Port=3
  FT2 Motor Output Shaft Torque : Outport  Port=4
  RT1 Info- Bus Signal : Outport  Port=5
  FT1 Info- Bus Signal : Outport  Port=6
  RT2 Info- Bus Signal : Outport  Port=7
  FT2 Info- Bus Signal : Outport  Port=8
  RT1 Battery Current Draw : Outport  Port=9
  FT1 Battery Current Draw : Outport  Port=10
  RT2 Battery Current Draw : Outport  Port=11
  FT2 Battery Current Draw : Outport  Port=12
  RT1 Motor Shaft Speed : Outport  Port=13
  FT1 Motor Shaft Speed : Outport  Port=14
  RT2 Motor Shaft Speed : Outport  Port=15
  FT2 Motor Shaft Speed : Outport  Port=16
  wires:
  Motor FT2/3 -> FT2 Motor Output Shaft Torque/1
  Battery Voltage Inport/1 -> Motor RT2/1, Motor FT2/1, Motor FT1/1, Motor RT1/1
  Motor RT1/1 -> RT1 Info- Bus Signal/1
  RT1 Motor Commanded Torque/1 -> Motor RT1/2
  "FT1 Motor Commanded Torque "/1 -> Motor FT1/2
  Motor RT2/1 -> RT2 Info- Bus Signal/1
  Motor FT1/1 -> FT1 Info- Bus Signal/1
  Motor FT2/1 -> FT2 Info- Bus Signal/1
  Motor FT1/4 -> FT1 Motor Shaft Speed/1
  FT2 Motor Commanded Torque/1 -> Motor FT2/2
  Motor RT2/4 -> RT2 Motor Shaft Speed/1
  Motor RT2/2 -> RT2 Battery Current Draw/1
  Motor FT2/4 -> FT2 Motor Shaft Speed/1
  Motor FT2/2 -> FT2 Battery Current Draw/1
  Motor RT1/3 -> RT1 Motor Output Shaft Torque/1
  RT2 Motor Commanded Torque/1 -> Motor RT2/2
  Motor RT1/4 -> RT1 Motor Shaft Speed/1
  Motor FT1/3 -> FT1 Motor Output Shaft Torque/1
  Motor RT2/3 -> RT2 Motor Output Shaft Torque/1
  Motor RT1/2 -> RT1 Battery Current Draw/1
  Motor FT1/2 -> FT1 Battery Current Draw/1
